simulink model "air_state_hopefully_final"  (R2017b)
settings: Solver=VariableStepAuto  StartTime=0.0  StopTime=10  RelTol=1e-3
settings Model: Creator=benma  LastModifiedBy=benma

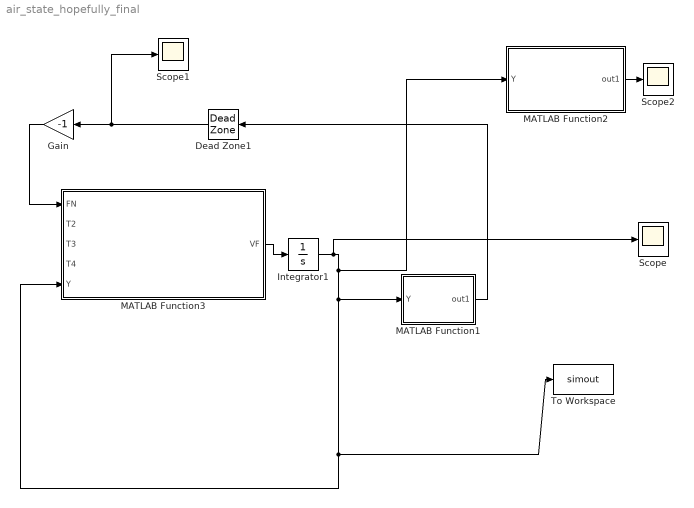
== system air_state_hopefully_final ==
  Dead Zone1 : DeadZone  LowerValue=-inf  UpperValue=0  SaturateOnIntegerOverflow=on
  Gain : Gain  Gain=-1
  Integrator1 : Integrator  InitialCondition=[130 270 80 330 0 0 0 0 0 0]*pi/180  ZeroCross=off
  MATLAB Function1 : MATLAB Function  TreatAsAtomicUnit=on
  MATLAB Function2 : MATLAB Function  TreatAsAtomicUnit=on
  MATLAB Function3 : MATLAB Function  TreatAsAtomicUnit=on
  Scope : Scope
  Scope1 : Scope
  Scope2 : Scope
  To Workspace : ToWorkspace  VariableName=simout  SaveFormat=Timeseries  SampleTime=-1
  wires:
  MATLAB Function2/1(out1) -> Scope2/1
  MATLAB Function3/1(VF) -> Integrator1/1
  Integrator1/1 -> Scope/1, MATLAB Function2/1(Y), MATLAB Function1/1(Y), To Workspace/1, MATLAB Function3/5(Y)
  MATLAB Function1/1(out1) -> Dead Zone1/1
  Dead Zone1/1 -> Scope1/1, Gain/1
  Gain/1 -> MATLAB Function3/1(FN)

== matlab function air_state_hopefully_final/MATLAB Function1 ==
  data: Y input; out1 output
function out1 = ground_force(Y)
%GROUND_FORCE
%    OUT1 = GROUND_FORCE(Y)

%    This function was generated by the Symbolic Math Toolbox version 8.0.
%    22-Oct-2018 11:02:05

if Y(5)<=0
    out1 = -100000*Y(5) - 100*Y(10);
else
    out1 = 0;

% t2 = Y(7);
% t3 = Y(1);
% t4 = Y(2);
% t5 = Y(6);
% t6 = Y(3);
% t7 = Y(8);
% t8 = Y(4);
% t9 = t3+t4+t6+t8;
% t10 = sin(t9);
% t11 = Y(9);
% t12 = t2+t5+t7+t11;
% t13 = t10.*t12.*(1.0./2.0);
% t14 = t3+t4;
% t15 = sin(t14);
% t16 = t2+t5;
% t17 = t15.*t16.*(5.0./2.0);
% t18 = t3+t4+t6; 
% t19 = sin(t18);
% t20 = t2+t5+t7;
% t21 = t19.*t20.*(3.0./2.0);
% out1 = -t7.*(t13+t21)-t5.*(t13+t17+t21+t5.*sin(t3).*(7.0./2.0))-t2.*(t13+t17+t21)-t10.*t11.*t12.*(1.0./2.0)+9.81e2./2.5e1;
end

== matlab function air_state_hopefully_final/MATLAB Function2 ==
  data: Y input; out1 output
function out1 = center_of_mass_state(Y)
%CENTER_OF_MASS_STATE
%    OUT1 = CENTER_OF_MASS_STATE(Y)

%    This function was generated by the Symbolic Math Toolbox version 8.0.
%    22-Oct-2018 12:19:55

t2 = Y(1);
t3 = Y(2);
t4 = Y(3);
t5 = t2+t3;
t6 = Y(4);
t7 = t2+t3+t4+t6;
t8 = t2+t3+t4;
t9 = sin(t2);
t10 = sin(t7);
t11 = Y(6);
t12 = sin(t5);
t13 = Y(7);
t14 = sin(t8);
t15 = Y(8);
t16 = cos(t2);
t17 = cos(t7);
t18 = Y(9);
t19 = t11+t13+t15+t18;
t20 = cos(t5);
t21 = t11+t13;
t22 = cos(t8);
t23 = t11+t13+t15;
out1 = [t16.*(7.0./8.0)+t17.*(1.0./8.0)+t20.*(5.0./8.0)+t22.*(3.0./8.0);t9.*(7.0./8.0)+t10.*(1.0./8.0)+t12.*(5.0./8.0)+t14.*(3.0./8.0)+Y(5);t9.*t11.*(-7.0./8.0)-t10.*t19.*(1.0./8.0)-t12.*t21.*(5.0./8.0)-t14.*t23.*(3.0./8.0);t11.*t16.*(7.0./8.0)+t17.*t19.*(1.0./8.0)+t20.*t21.*(5.0./8.0)+t22.*t23.*(3.0./8.0)+Y(10)];

== matlab function air_state_hopefully_final/MATLAB Function3 ==
  data: FN input; T2 input; VF output; T3 input; T4 input; Y input
function VF = Air_with_force(FN,T2,T3,T4,Y)
%AIR_WITH_FORCE
%    VF = AIR_WITH_FORCE(FN,T2,T3,T4,Y)

%    This function was generated by the Symbolic Math Toolbox version 8.0.
%    27-Oct-2018 21:34:20

t2 = Y(1);
t3 = t2.*2.0;
t4 = Y(2);
t5 = t4.*2.0;
t6 = Y(4);
t7 = Y(3);
t8 = t7.*2.0;
t9 = t6.*2.0;
t10 = Y(6);
t11 = t10.^2;
t12 = t3+t4+t7+t9;
t13 = cos(t12);
t14 = t3+t4;
t15 = sin(t14);
t16 = Y(7);
t17 = t4-t7;
t18 = sin(t17);
t19 = t16.^2;
t20 = Y(8);
t21 = t4+t8;
t22 = sin(t21);
t23 = t4-t9;
t24 = sin(t23);
t25 = t4+t9;
t26 = sin(t25);
t27 = cos(t8);
t28 = cos(t9);
t29 = t3+t4-t7;
t30 = sin(t29);
t31 = t20.^2;
t32 = t3+t4+t8;
t33 = sin(t32);
t34 = t3+t4-t9;
t35 = sin(t34);
t36 = t3+t4+t9;
t37 = sin(t36);
t38 = -t4+t7+t9;
t39 = sin(t38);
t40 = t4+t8+t9;
t41 = sin(t40);
t42 = cos(t14);
t43 = cos(t21);
t44 = cos(t17);
t45 = cos(t23);
t46 = cos(t25);
t47 = t3+t4-t6-t7;
t48 = sin(t47);
t49 = t3+t4-t7-t9;
t50 = sin(t49);
t51 = Y(9);
t52 = t3+t4+t8+t9;
t53 = sin(t52);
t54 = cos(t32);
t55 = cos(t29);
t56 = cos(t34);
t57 = cos(t36);
t58 = cos(t40);
t59 = cos(t38);
t60 = cos(t52);
t61 = cos(t49);
t62 = t3-t8;
t63 = t3+t8;
t64 = t3-t9;
t65 = t3+t9;
t66 = t5+t8;
t67 = t5-t9;
t68 = t5+t9;
t69 = t3+t4+t6+t7;
t70 = sin(t69);
t71 = t51.^2;
t72 = -t3+t8+t9;
t73 = t3+t8+t9;
t74 = t5+t8+t9;
t75 = sin(t4);
t76 = t3+t5;
t77 = cos(t76);
t78 = t8+t9;
t79 = cos(t78);
t80 = t4+t7;
t81 = sin(t80);
t82 = t3+t5+t8;
t83 = cos(t82);
t84 = t3+t5+t9;
t85 = cos(t84);
t86 = cos(t4);
t87 = t3+t4+t7;
t88 = sin(t87);
t89 = -t4+t6+t7;
t90 = sin(t89);
t91 = t4+t6-t7;
t92 = sin(t91);
t93 = t4-t6+t7;
t94 = sin(t93);
t95 = t4+t7+t9;
t96 = sin(t95);
t97 = t3+t5+t8+t9;
t98 = cos(t97);
t99 = cos(t80);
t100 = t3+t4+t6-t7;
t101 = t3+t4-t6+t7;
t102 = sin(t100);
t103 = sin(t101);
t104 = sin(t12);
t105 = cos(t87);
t106 = cos(t95);
t107 = t3+t5-t9;
t108 = cos(t107);
t109 = cos(t72);
t110 = cos(t73);
t111 = cos(t74);
t112 = t98.*3.0;
t113 = cos(t3);
t114 = cos(t5);
t115 = t77.*2.19e2;
t116 = cos(t62);
t117 = t116.*2.43e2;
t118 = cos(t63);
t119 = t118.*2.43e2;
t120 = cos(t64);
t121 = t120.*2.16e2;
t122 = cos(t65);
t123 = t122.*2.16e2;
t124 = cos(t66);
t125 = t124.*8.1e1;
t126 = cos(t67);
t127 = t126.*8.1e1;
t128 = cos(t68);
t129 = t128.*8.1e1;
t130 = t79.*8.1e1;
t131 = sin(t3);
t132 = sin(t5);
t133 = sin(t8);
t134 = T3.*t13.*9.0;
t135 = cos(t100);
t136 = cos(t101);
t137 = T4.*t136.*2.7e1;
t138 = t11.*t18.*1.08e2;
t139 = t3+t7;
t140 = sin(t139);
t141 = t18.*t19.*1.08e2;
t142 = t18.*t31.*1.08e2;
t143 = t5+t7;
t144 = sin(t143);
t145 = -t6+t7;
t146 = sin(t145);
t147 = t7+t9;
t148 = sin(t147);
t149 = t3+t5+t7;
t150 = sin(t149);
t151 = t19.*t33.*(2.7e1./2.0);
t152 = t3+t6-t7;
t153 = sin(t152);
t154 = t19.*t35.*1.8e1;
t155 = t19.*t37.*1.8e1;
t156 = t3-t6+t7;
t157 = sin(t156);
t158 = t11.*t39.*9.0;
t159 = -t3+t7+t9;
t160 = sin(t159);
t161 = t3+t7+t9;
t162 = sin(t161);
t163 = t19.*t39.*9.0;
t164 = t5-t6+t7;
t165 = sin(t164);
t166 = t31.*t39.*9.0;
t167 = t5+t7+t9;
t168 = sin(t167);
t169 = t19.*t41.*3.0;
t170 = t2+t5;
t171 = cos(t170);
t172 = t2-t8;
t173 = cos(t172);
t174 = t2+t8;
t175 = cos(t174);
t176 = t2-t9;
t177 = cos(t176);
t178 = t2+t9;
t179 = cos(t178);
t180 = T3.*t42.*4.11e2;
t181 = T3.*t43.*1.62e2;
t182 = cos(t139);
t183 = T4.*t44.*3.24e2;
t184 = T3.*t45.*8.1e1;
t185 = T3.*t46.*8.1e1;
t186 = cos(t143);
t187 = cos(t147);
t188 = t11.*t50.*(9.0./2.0);
t189 = t3+t5-t6+t7;
t190 = sin(t189);
t191 = t19.*t50.*(9.0./2.0);
t192 = t31.*t50.*(9.0./2.0);
t193 = t3+t5+t7+t9;
t194 = sin(t193);
t195 = t2+t5+t8;
t196 = cos(t195);
t197 = FN.*t196.*2.7e1;
t198 = t2+t5-t9;
t199 = cos(t198);
t200 = FN.*t199.*2.7e1;
t201 = t2+t5+t9;
t202 = cos(t201);
t203 = FN.*t202.*2.7e1;
t204 = t2+t8+t9;
t205 = cos(t204);
t206 = FN.*t205.*9.0;
t207 = T3.*t55.*1.62e2;
t208 = cos(t149);
t209 = T3.*t59.*5.4e1;
t210 = cos(t159);
t211 = cos(t161);
t212 = cos(t167);
t213 = t2+t5+t8+t9;
t214 = cos(t213);
t215 = cos(t47);
t216 = T4.*t215.*3.6e1;
t217 = T3.*t60.*9.0;
t218 = T4.*t61.*2.7e1;
t219 = cos(t193);
t220 = sin(t76);
t221 = t3-t7;
t222 = sin(t221);
t223 = sin(t63);
t224 = sin(t62);
t225 = sin(t64);
t226 = t11.*t225.*3.6e1;
t227 = sin(t65);
t228 = t11.*t227.*3.6e1;
t229 = sin(t66);
t230 = sin(t67);
t231 = sin(t68);
t232 = sin(t78);
t233 = t11.*t70.*(1.0./2.0);
t234 = t19.*t70.*(1.0./2.0);
t235 = t31.*t70.*(1.0./2.0);
t236 = t70.*t71.*(1.0./2.0);
t237 = sin(t107);
t238 = sin(t84);
t239 = sin(t73);
t240 = sin(t72);
t241 = sin(t74);
t242 = t11.*t241.*(3.0./2.0);
t243 = t4+t6+t7;
t244 = cos(t243);
t245 = T4.*t244.*1.8e1;
t246 = t19.*t75.*(6.75e2./2.0);
t247 = sin(t7);
t248 = cos(t221);
t249 = T2.*t79.*2.7e1;
t250 = -t2+t8+t9;
t251 = cos(t250);
t252 = FN.*t251.*9.0;
t253 = cos(t69);
t254 = t11.*t81.*4.5e1;
t255 = t19.*t81.*4.5e1;
t256 = t31.*t81.*4.5e1;
t257 = t6+t7;
t258 = sin(t257);
t259 = T2.*t108.*2.7e1;
t260 = T2.*t85.*2.7e1;
t261 = cos(t2);
t262 = FN.*t261.*4.93e2;
t263 = cos(t7);
t264 = t11.*t92.*2.7e1;
t265 = t11.*t94.*(2.7e1./2.0);
t266 = -t3+t6+t7;
t267 = sin(t266);
t268 = t3+t6+t7;
t269 = sin(t268);
t270 = t19.*t92.*2.7e1;
t271 = t19.*t94.*(2.7e1./2.0);
t272 = t31.*t92.*2.7e1;
t273 = t31.*t94.*(2.7e1./2.0);
t274 = t5+t6+t7;
t275 = sin(t274);
t276 = t71.*t92.*2.7e1;
t277 = t71.*t94.*(2.7e1./2.0);
t278 = T3.*t99.*2.16e2;
t279 = t3+t5+t6+t7;
t280 = t11.*t104.*(3.0./2.0);
t281 = sin(t279);
t282 = t19.*t104.*(3.0./2.0);
t283 = t31.*t104.*(3.0./2.0);
t284 = T4.*t105.*8.1e1;
t285 = cos(t89);
t286 = cos(t91);
t287 = T4.*t286.*1.62e2;
t288 = cos(t93);
t289 = T4.*t106.*2.7e1;
t290 = t10.*t16.*t81.*9.0e1;
t291 = t10.*t20.*t81.*9.0e1;
t292 = t16.*t20.*t81.*9.0e1;
t293 = t10.*t16.*t92.*5.4e1;
t294 = t10.*t16.*t94.*2.7e1;
t295 = t10.*t20.*t92.*5.4e1;
t296 = t10.*t20.*t94.*2.7e1;
t297 = t10.*t51.*t92.*5.4e1;
t298 = t16.*t20.*t92.*5.4e1;
t299 = t10.*t51.*t94.*2.7e1;
t300 = t16.*t20.*t94.*2.7e1;
t301 = t16.*t51.*t92.*5.4e1;
t302 = t16.*t51.*t94.*2.7e1;
t303 = t20.*t51.*t92.*5.4e1;
t304 = t20.*t51.*t94.*2.7e1;
t305 = t10.*t16.*t104.*3.0;
t306 = t10.*t20.*t104.*3.0;
t307 = t16.*t20.*t104.*3.0;
t308 = t10.*t16.*t18.*2.16e2;
t309 = t10.*t18.*t20.*2.16e2;
t310 = t16.*t18.*t20.*2.16e2;
t311 = t10.*t16.*t33.*2.7e1;
t312 = t10.*t16.*t35.*3.6e1;
t313 = t10.*t16.*t37.*3.6e1;
t314 = t10.*t16.*t39.*1.8e1;
t315 = t10.*t20.*t39.*1.8e1;
t316 = t10.*t16.*t41.*6.0;
t317 = t16.*t20.*t39.*1.8e1;
t318 = t10.*t16.*t50.*9.0;
t319 = t10.*t20.*t50.*9.0;
t320 = t16.*t20.*t50.*9.0;
t321 = t10.*t16.*t70;
t322 = t10.*t20.*t70;
t323 = t10.*t51.*t70;
t324 = t16.*t20.*t70;
t325 = t16.*t51.*t70;
t326 = t20.*t51.*t70;
t327 = t10.*t16.*t75.*6.75e2;
t493 = t83.*2.7e1;
t494 = t108.*2.7e1;
t495 = t85.*2.7e1;
t496 = t109.*2.7e1;
t497 = t110.*2.7e1;
t498 = t111.*9.0;
t499 = t113.*1.725e3;
t500 = t114.*6.57e2;
t501 = t27.*7.29e2;
t502 = t28.*6.39e2;
t328 = t112+t115+t117+t119+t121+t123+t125+t127+t129+t130-t493-t494-t495-t496-t497-t498-t499-t500-t501-t502+2.542e3;
t329 = 1.0./t328;
t330 = t11.*t132.*(2.19e2./2.0);
t331 = sin(t9);
t332 = t2+t4+t8+t9;
t333 = cos(t332);
t334 = FN.*t333.*6.0;
t335 = cos(t279);
t336 = T4.*t335.*1.2e1;
t337 = t3+t6;
t338 = sin(t337);
t339 = t11.*t146.*(1.53e2./2.0);
t340 = t5+t6;
t341 = sin(t340);
t342 = t19.*t146.*(1.53e2./2.0);
t343 = t31.*t146.*(1.53e2./2.0);
t344 = t6+t8;
t345 = sin(t344);
t346 = t71.*t146.*(1.53e2./2.0);
t347 = T2.*t113.*7.41e2;
t348 = t11.*t33.*(2.7e1./2.0);
t349 = t11.*t153.*2.7e1;
t350 = t31.*t150.*1.8e1;
t351 = t3+t5+t6;
t352 = sin(t351);
t353 = t19.*t153.*2.7e1;
t354 = t31.*t153.*2.7e1;
t355 = -t3+t6+t8;
t356 = sin(t355);
t357 = t3+t6+t8;
t358 = sin(t357);
t359 = t71.*t153.*2.7e1;
t360 = t31.*t160.*9.0;
t361 = t31.*t162.*9.0;
t362 = t5+t6+t8;
t363 = sin(t362);
t364 = t31.*t168.*(9.0./2.0);
t365 = t2-t4;
t366 = cos(t365);
t367 = T4.*t182.*2.43e2;
t368 = T4.*t186.*1.62e2;
t369 = cos(t145);
t370 = T4.*t187.*1.53e2;
t371 = t11.*t190.*(9.0./2.0);
t372 = t19.*t190.*(9.0./2.0);
t373 = t31.*t190.*(9.0./2.0);
t374 = t3+t5+t6+t8;
t375 = sin(t374);
t376 = t71.*t190.*(9.0./2.0);
t377 = -t2+t4+t8;
t378 = cos(t377);
t379 = FN.*t378.*8.1e1;
t380 = -t2+t4+t9;
t381 = cos(t380);
t382 = FN.*t381.*5.4e1;
t383 = t2-t4+t9;
t384 = cos(t383);
t385 = FN.*t384.*5.4e1;
t386 = T2.*t54.*8.1e1;
t387 = T2.*t56.*5.4e1;
t388 = T2.*t57.*5.4e1;
t389 = T2.*t58.*1.8e1;
t390 = cos(t152);
t391 = T4.*t390.*1.62e2;
t392 = cos(t156);
t393 = T4.*t392.*1.62e2;
t394 = cos(t164);
t395 = T4.*t394.*8.1e1;
t396 = -t2+t4+t8+t9;
t397 = cos(t396);
t398 = cos(t189);
t399 = T4.*t219.*9.0;
t400 = t11.*t220.*(7.3e1./2.0);
t401 = t19.*t220.*(7.3e1./2.0);
t402 = t31.*t222.*(2.43e2./2.0);
t403 = t3-t6;
t404 = sin(t403);
t405 = t11.*t229.*(2.7e1./2.0);
t406 = t5-t6;
t407 = sin(t406);
t408 = t11.*t231.*2.7e1;
t409 = sin(t82);
t410 = t3+t5-t6;
t411 = sin(t410);
t412 = t11.*t240.*(9.0./2.0);
t413 = t19.*t240.*(9.0./2.0);
t414 = t19.*t239.*(9.0./2.0);
t415 = t31.*t247.*(6.93e2./2.0);
t416 = sin(t6);
t417 = T2.*t124.*8.1e1;
t418 = T4.*t248.*2.43e2;
t419 = T3.*t120.*1.08e2;
t420 = T3.*t122.*1.08e2;
t421 = t11.*t258.*(6.1e1./2.0);
t422 = t19.*t258.*(6.1e1./2.0);
t423 = t31.*t258.*(6.1e1./2.0);
t424 = t71.*t258.*(6.1e1./2.0);
t425 = T2.*t83.*2.7e1;
t426 = T3.*t83.*2.7e1;
t427 = T2.*t86.*6.03e2;
t428 = t11.*t88.*(2.7e1./2.0);
t429 = t11.*t96.*(9.0./2.0);
t430 = t2+t4;
t431 = cos(t430);
t432 = FN.*t431.*3.47e2;
t433 = cos(t257);
t434 = T4.*t433.*2.85e2;
t435 = t11.*t281;
t436 = t19.*t281;
t437 = t31.*t281;
t438 = t71.*t281;
t439 = t2+t4+t8;
t440 = cos(t439);
t441 = t2+t4-t9;
t442 = cos(t441);
t443 = t2+t4+t9;
t444 = cos(t443);
t445 = cos(t266);
t446 = cos(t268);
t447 = cos(t274);
t448 = t10.*t16.*t258.*6.1e1;
t449 = t10.*t20.*t258.*6.1e1;
t450 = t10.*t51.*t258.*6.1e1;
t451 = t16.*t20.*t258.*6.1e1;
t452 = t16.*t51.*t258.*6.1e1;
t453 = t20.*t51.*t258.*6.1e1;
t454 = t10.*t16.*t281.*2.0;
t455 = t10.*t20.*t281.*2.0;
t456 = t10.*t51.*t281.*2.0;
t457 = t16.*t20.*t281.*2.0;
t458 = t16.*t51.*t281.*2.0;
t459 = t20.*t51.*t281.*2.0;
t460 = t10.*t16.*t146.*1.53e2;
t461 = t10.*t20.*t146.*1.53e2;
t462 = t10.*t51.*t146.*1.53e2;
t463 = t16.*t20.*t146.*1.53e2;
t464 = t16.*t51.*t146.*1.53e2;
t465 = t20.*t51.*t146.*1.53e2;
t466 = t10.*t20.*t150.*3.6e1;
t467 = t10.*t16.*t153.*5.4e1;
t468 = t16.*t20.*t150.*3.6e1;
t469 = t10.*t20.*t153.*5.4e1;
t470 = t10.*t51.*t153.*5.4e1;
t471 = t16.*t20.*t153.*5.4e1;
t472 = t10.*t20.*t160.*1.8e1;
t473 = t10.*t20.*t162.*1.8e1;
t474 = t16.*t51.*t153.*5.4e1;
t475 = t16.*t20.*t160.*1.8e1;
t476 = t16.*t20.*t162.*1.8e1;
t477 = t10.*t20.*t168.*9.0;
t478 = t20.*t51.*t153.*5.4e1;
t479 = t16.*t20.*t168.*9.0;
t480 = t10.*t16.*t190.*9.0;
t481 = t10.*t20.*t190.*9.0;
t482 = t10.*t51.*t190.*9.0;
t483 = t16.*t20.*t190.*9.0;
t484 = t16.*t51.*t190.*9.0;
t485 = t20.*t51.*t190.*9.0;
t486 = t10.*t16.*t220.*7.3e1;
t487 = t10.*t20.*t222.*2.43e2;
t488 = t16.*t20.*t222.*2.43e2;
t489 = t10.*t16.*t240.*9.0;
t490 = t10.*t16.*t239.*9.0;
t491 = t10.*t20.*t247.*6.93e2;
t492 = t16.*t20.*t247.*6.93e2;
t503 = t11.*t133.*(2.43e2./2.0);
t504 = t19.*t133.*(2.43e2./2.0);
t505 = -t2+t4+t7+t9;
t506 = cos(t505);
t507 = FN.*t506.*9.0;
t508 = t2-t4+t7+t9;
t509 = cos(t508);
t510 = t2+t4-t7-t9;
t511 = cos(t510);
t512 = FN.*t511.*1.8e1;
t513 = T3.*t114.*3.15e2;
t514 = t11.*t39.*1.8e1;
t515 = t11.*t165.*(2.7e1./2.0);
t516 = t19.*t165.*(2.7e1./2.0);
t517 = t11.*t168.*(9.0./2.0);
t518 = t71.*t352.*(2.1e1./2.0);
t519 = t19.*t168.*(9.0./2.0);
t520 = t71.*t356.*(2.7e1./2.0);
t521 = t71.*t358.*(2.7e1./2.0);
t522 = t71.*t363.*(9.0./2.0);
t523 = T2.*t44.*3.24e2;
t524 = cos(t337);
t525 = cos(t340);
t526 = cos(t344);
t527 = T2.*t208.*5.4e1;
t528 = T3.*t208.*5.4e1;
t529 = T2.*t210.*5.4e1;
t530 = T2.*t211.*5.4e1;
t531 = cos(t351);
t532 = T2.*t212.*2.7e1;
t533 = cos(t355);
t534 = T3.*t210.*5.4e1;
t535 = cos(t357);
t536 = T3.*t211.*5.4e1;
t537 = cos(t362);
t538 = T3.*t212.*2.7e1;
t539 = T2.*t61.*2.7e1;
t540 = cos(t374);
t541 = t11.*t222.*(2.43e2./2.0);
t542 = t19.*t222.*(2.43e2./2.0);
t543 = t11.*t224.*(8.1e1./2.0);
t544 = t11.*t223.*(8.1e1./2.0);
t545 = t19.*t224.*(8.1e1./2.0);
t546 = t31.*t223.*(8.1e1./2.0);
t547 = t19.*t229.*(2.7e1./2.0);
t548 = t11.*t230.*2.7e1;
t549 = t71.*t404.*(1.59e2./2.0);
t550 = t31.*t229.*(2.7e1./2.0);
t551 = t11.*t232.*(2.7e1./2.0);
t552 = t71.*t407.*(6.3e1./2.0);
t553 = t19.*t232.*(2.7e1./2.0);
t554 = t11.*t238.*9.0;
t555 = t19.*t238.*9.0;
t556 = t2+t4+t7;
t557 = cos(t556);
t558 = FN.*t557.*3.6e1;
t559 = t71.*t416.*(4.67e2./2.0);
t560 = cos(t403);
t561 = cos(t406);
t562 = T3.*t79.*8.1e1;
t563 = sin(t97);
t564 = t2+t4+t7+t9;
t565 = cos(t564);
t566 = cos(t410);
t567 = T3.*t111.*9.0;
t568 = T4.*t109.*2.7e1;
t569 = T4.*t110.*2.7e1;
t570 = T4.*t111.*9.0;
t571 = T2.*t263.*6.75e2;
t572 = T3.*t263.*6.75e2;
t573 = cos(t6);
t574 = t11.*t102.*(2.7e1./2.0);
t575 = t11.*t103.*(9.0./2.0);
t576 = -t2+t4+t7;
t577 = cos(t576);
t578 = t2-t4+t7;
t579 = cos(t578);
t580 = FN.*t579.*1.62e2;
t581 = t2+t4-t7;
t582 = cos(t581);
t583 = T2.*t105.*8.1e1;
t584 = T2.*t106.*2.7e1;
t585 = t10.*t16.*t133.*2.43e2;
t586 = t10.*t16.*t165.*2.7e1;
t587 = t10.*t51.*t352.*2.1e1;
t588 = t10.*t16.*t168.*9.0;
t589 = t16.*t51.*t352.*2.1e1;
t590 = t10.*t51.*t356.*2.7e1;
t591 = t10.*t51.*t358.*2.7e1;
t592 = t20.*t51.*t352.*2.1e1;
t593 = t16.*t51.*t356.*2.7e1;
t594 = t16.*t51.*t358.*2.7e1;
t595 = t10.*t51.*t363.*9.0;
t596 = t20.*t51.*t356.*2.7e1;
t597 = t20.*t51.*t358.*2.7e1;
t598 = t16.*t51.*t363.*9.0;
t599 = t20.*t51.*t363.*9.0;
t600 = t10.*t16.*t222.*2.43e2;
t601 = t10.*t16.*t224.*8.1e1;
t602 = t10.*t20.*t223.*8.1e1;
t603 = t10.*t16.*t229.*2.7e1;
t604 = t16.*t20.*t223.*8.1e1;
t605 = t10.*t51.*t404.*1.59e2;
t606 = t10.*t20.*t229.*2.7e1;
t607 = t16.*t51.*t404.*1.59e2;
t608 = t16.*t20.*t229.*2.7e1;
t609 = t10.*t51.*t407.*6.3e1;
t610 = t10.*t16.*t232.*2.7e1;
t611 = t20.*t51.*t404.*1.59e2;
t612 = t16.*t51.*t407.*6.3e1;
t613 = t20.*t51.*t407.*6.3e1;
t614 = t10.*t16.*t238.*1.8e1;
t615 = t10.*t51.*t416.*4.67e2;
t616 = t16.*t51.*t416.*4.67e2;
t617 = t20.*t51.*t416.*4.67e2;
t618 = t2-t4+t6-t7;
t619 = cos(t618);
t620 = t2-t4-t6+t7;
t621 = cos(t620);
t622 = t2+t4-t6-t7;
t623 = cos(t622);
t624 = sin(t365);
t625 = t2+t4+t6+t7;
t626 = sin(t625);
t627 = sin(t377);
t628 = sin(t380);
t629 = sin(t383);
t630 = sin(t396);
t631 = cos(t625);
t632 = sin(t556);
t633 = -t2+t4+t6+t7;
t634 = t2-t4+t6+t7;
t635 = t2+t4+t6-t7;
t636 = t2+t4-t6+t7;
t637 = sin(t633);
t638 = sin(t634);
t639 = sin(t635);
t640 = sin(t636);
t641 = sin(t564);
t642 = cos(t633);
t643 = cos(t634);
t644 = cos(t635);
t645 = cos(t636);
t646 = sin(t430);
t647 = sin(t576);
t648 = sin(t578);
t649 = sin(t581);
t650 = sin(t439);
t651 = sin(t441);
t652 = sin(t443);
t653 = sin(t618);
t654 = sin(t620);
t655 = sin(t622);
t656 = sin(t505);
t657 = sin(t508);
t658 = sin(t510);
t659 = sin(t332);
VF = [t10;t16;t20;t51;Y(10);(T2.*3.972e3+t134.*6.0+t137.*6.0+t138.*6.0+t141.*6.0+t142.*6.0+t151.*6.0+t154.*6.0+t155.*6.0+t158.*6.0+t163.*6.0+t166.*6.0+t169.*6.0+t180.*6.0+t181.*6.0+t183.*6.0+t184.*6.0+t185.*6.0+t188.*6.0+t191.*6.0+t192.*6.0+t197.*6.0+t200.*6.0+t203.*6.0+t206.*6.0+t207.*6.0+t209.*6.0+t216.*6.0+t217.*6.0+t218.*6.0+t226.*6.0+t228.*6.0+t233.*6.0+t234.*6.0+t235.*6.0+t236.*6.0+t242.*6.0+t245.*6.0+t246.*6.0+t249.*6.0+t252.*6.0+t254.*6.0+t255.*6.0+t256.*6.0+t259.*6.0+t260.*6.0+t262.*6.0+t264.*6.0+t265.*6.0+t270.*6.0+t271.*6.0+t272.*6.0+t273.*6.0+t276.*6.0+t277.*6.0+t278.*6.0+t280.*6.0+t282.*6.0+t283.*6.0+t284.*6.0+t287.*6.0+t289.*6.0+t290.*6.0+t291.*6.0+t292.*6.0+t293.*6.0+t294.*6.0+t295.*6.0+t296.*6.0+t297.*6.0+t298.*6.0+t299.*6.0+t300.*6.0+t301.*6.0+t302.*6.0+t303.*6.0+t304.*6.0+t305.*6.0+t306.*6.0+t307.*6.0+t308.*6.0+t309.*6.0+t310.*6.0+t311.*6.0+t312.*6.0+t313.*6.0+t314.*6.0+t315.*6.0+t316.*6.0+t317.*6.0+t318.*6.0+t319.*6.0+t320.*6.0+t321.*6.0+t322.*6.0+t323.*6.0+t324.*6.0+t325.*6.0+t326.*6.0+t327.*6.0+t330.*6.0+t348.*6.0+t386.*6.0+t387.*6.0+t388.*6.0+t389.*6.0+t412.*6.0+t425.*6.0+t427.*6.0+t543.*6.0+t544.*6.0-FN.*t171.*1.314e3-FN.*t173.*4.86e2-FN.*t175.*4.86e2-FN.*t177.*3.78e2-FN.*t179.*3.78e2-FN.*t214.*1.8e1-T4.*t13.*5.4e1-T2.*t27.*1.458e3-T2.*t28.*1.026e3-T2.*t42.*2.466e3-T2.*t43.*9.72e2-T2.*t45.*4.86e2-T3.*t44.*1.944e3-T2.*t46.*4.86e2-T3.*t54.*4.86e2-T3.*t56.*3.24e2-T4.*t55.*9.72e2-T3.*t57.*3.24e2-T3.*t58.*1.08e2-T2.*t60.*5.4e1-T4.*t59.*3.24e2-T3.*t61.*1.62e2-T2.*t77.*1.314e3-T3.*t86.*3.618e3-T2.*t98.*1.8e1-T4.*t99.*1.296e3-T3.*t105.*4.86e2-T3.*t106.*1.62e2-T4.*t135.*4.86e2-T4.*t253.*1.8e1-T4.*t285.*4.32e2-T4.*t288.*4.86e2-t11.*t15.*9.03e2-t11.*t22.*1.62e2-t15.*t19.*9.03e2-t11.*t24.*2.43e2-t11.*t26.*2.43e2-t11.*t30.*3.24e2-t19.*t22.*1.62e2-t19.*t24.*2.43e2-t19.*t26.*2.43e2+t11.*t35.*1.08e2+t11.*t37.*1.08e2-t19.*t30.*3.24e2+t11.*t41.*1.8e1-t11.*t48.*1.8e1-t30.*t31.*3.24e2-t11.*t53.*9.0-t19.*t48.*1.8e1-t19.*t53.*9.0-t31.*t48.*1.8e1+t11.*t75.*2.025e3-t11.*t88.*8.1e1-t11.*t90.*3.6e1-t11.*t96.*2.7e1-t19.*t88.*8.1e1-t19.*t90.*3.6e1-t11.*t102.*8.1e1-t11.*t103.*2.7e1-t19.*t96.*2.7e1-t31.*t88.*8.1e1-t48.*t71.*1.8e1-t19.*t102.*8.1e1-t31.*t90.*3.6e1-t19.*t103.*2.7e1-t31.*t96.*2.7e1-t31.*t102.*8.1e1-t31.*t103.*2.7e1-t11.*t131.*1.725e3-t71.*t90.*3.6e1-t71.*t102.*8.1e1-t71.*t103.*2.7e1-t11.*t229.*8.1e1-t11.*t230.*8.1e1-t11.*t231.*8.1e1-t11.*t239.*2.7e1-t10.*t15.*t16.*1.806e3-t10.*t16.*t22.*3.24e2-t10.*t16.*t24.*4.86e2-t10.*t16.*t26.*4.86e2-t10.*t16.*t30.*6.48e2-t10.*t20.*t30.*6.48e2-t16.*t20.*t30.*6.48e2-t10.*t16.*t48.*3.6e1-t10.*t20.*t48.*3.6e1-t10.*t16.*t53.*1.8e1-t16.*t20.*t48.*3.6e1-t10.*t48.*t51.*3.6e1-t10.*t16.*t88.*1.62e2-t16.*t48.*t51.*3.6e1-t10.*t16.*t90.*7.2e1-t10.*t20.*t88.*1.62e2-t20.*t48.*t51.*3.6e1-t10.*t20.*t90.*7.2e1-t10.*t16.*t96.*5.4e1-t16.*t20.*t88.*1.62e2-t10.*t20.*t96.*5.4e1-t16.*t20.*t90.*7.2e1-t10.*t16.*t102.*1.62e2-t10.*t16.*t103.*5.4e1-t10.*t20.*t102.*1.62e2-t16.*t20.*t96.*5.4e1-t10.*t20.*t103.*5.4e1-t16.*t20.*t102.*1.62e2-t16.*t20.*t103.*5.4e1-t10.*t51.*t90.*7.2e1-t16.*t51.*t90.*7.2e1-t20.*t51.*t90.*7.2e1-t10.*t51.*t102.*1.62e2-t10.*t51.*t103.*5.4e1-t16.*t51.*t102.*1.62e2-t16.*t51.*t103.*5.4e1-t20.*t51.*t102.*1.62e2-t20.*t51.*t103.*5.4e1)./(t27.*-7.29e2-t28.*6.39e2-t83.*2.7e1-t85.*2.7e1-t109.*2.7e1-t110.*2.7e1-t111.*9.0+t112-t113.*1.725e3-t114.*6.57e2+t115+t117+t119+t121+t123+t125+t127+t129+t130-cos(t3+t5-t6.*2.0).*2.7e1+2.542e3);t329.*(T2.*-1.6e3+T3.*9.38e2-t134-t137-t138-t141-t142-t151-t154-t155-t158-t163-t166-t169-t180-t181-t183-t184-t185-t188-t191-t192-t197-t200-t203-t206-t207-t209-t216-t217-t218-t226-t228-t233-t234-t235-t236-t242-t245-t246-t249-t252-t254-t255-t256-t259-t260-t262-t264-t265-t270-t271-t272-t273-t276-t277-t278-t280-t282-t283-t284-t287-t289-t290-t291-t292-t293-t294-t295-t296-t297-t298-t299-t300-t301-t302-t303-t304-t305-t306-t307-t308-t309-t310-t311-t312-t313-t314-t315-t316-t317-t318-t319-t320-t321-t322-t323-t324-t325-t326-t327+t334+t336+t339+t342+t343+t346+t347+t349+t350+t353+t354+t359+t360+t361+t364+t367+t368+t370+t371+t372+t373+t376+t379+t382+t385+t391+t393+t395+t399+t400+t401+t402+t405+t408+t413+t414+t415+t417+t418+t419+t420+t421+t422+t423+t424+t426+t428+t429+t432+t434+t435+t436+t437+t438+t448+t449+t450+t451+t452+t453+t454+t455+t456+t457+t458+t459+t460+t461+t462+t463+t464+t465+t466+t467+t468+t469+t470+t471+t472+t473+t474+t475+t476+t477+t478+t479+t480+t481+t482+t483+t484+t485+t486+t487+t488+t489+t490+t491+t492+t503+t504+t517+t519+t528+t534+t536+t538+t541+t542+t545+t548+t567+t572+t574+t575+t585+t588+t600+t601+FN.*t171.*2.19e2+FN.*t173.*8.1e1+FN.*t175.*8.1e1+FN.*t177.*6.3e1+FN.*t179.*6.3e1+FN.*t214.*3.0-FN.*t366.*4.11e2-FN.*t397.*9.0-FN.*t440.*5.4e1-FN.*t442.*4.5e1-FN.*t444.*4.5e1+T4.*t13.*9.0+T2.*t27.*2.43e2+T2.*t28.*4.5e2-T3.*t28.*2.79e2+T2.*t42.*8.22e2+T2.*t43.*3.24e2+T2.*t45.*1.62e2+T3.*t44.*3.24e2+T2.*t46.*1.62e2-T2.*t54.*1.62e2+T3.*t54.*8.1e1-T2.*t56.*1.08e2-T2.*t57.*1.08e2+T3.*t56.*5.4e1+T4.*t55.*1.62e2-T2.*t58.*3.6e1+T3.*t57.*5.4e1+T3.*t58.*1.8e1+T2.*t60.*1.8e1+T4.*t59.*5.4e1+T3.*t61.*2.7e1+T2.*t77.*2.19e2-T2.*t83.*5.4e1-T2.*t86.*1.206e3+T3.*t86.*6.03e2+T2.*t98.*6.0-T3.*t98.*3.0+T4.*t99.*2.16e2+T3.*t105.*8.1e1+T3.*t106.*2.7e1-T2.*t111.*9.0-T3.*t113.*7.41e2-T2.*t120.*1.08e2-T2.*t122.*1.08e2-T3.*t124.*8.1e1+T4.*t135.*8.1e1-T3.*t182.*2.43e2-T3.*t186.*1.62e2-T3.*t187.*1.53e2-T4.*t208.*5.4e1-T4.*t210.*5.4e1-T4.*t211.*5.4e1-T4.*t212.*2.7e1-T3.*t219.*9.0-T3.*t248.*2.43e2+T4.*t253.*3.0-T4.*t263.*6.75e2+T4.*t285.*7.2e1+T4.*t288.*8.1e1-T4.*t369.*4.59e2-T4.*t398.*2.7e1-T4.*t445.*9.9e1-T4.*t446.*9.9e1-T4.*t447.*3.6e1+t11.*t15.*2.19e2+t11.*t22.*8.1e1+t15.*t19.*(3.01e2./2.0)+t11.*t24.*8.1e1+t11.*t26.*8.1e1+t11.*t30.*5.4e1+t19.*t22.*2.7e1+t19.*t24.*(8.1e1./2.0)-t11.*t33.*2.7e1+t19.*t26.*(8.1e1./2.0)-t11.*t35.*2.7e1-t11.*t37.*2.7e1+t19.*t30.*5.4e1-t11.*t41.*9.0+t11.*t48.*3.0+t30.*t31.*5.4e1+t11.*t53.*3.0+t19.*t48.*3.0+t19.*t53.*(3.0./2.0)+t31.*t48.*3.0-t11.*t75.*6.48e2+t11.*t90.*6.0+t19.*t88.*(2.7e1./2.0)+t19.*t90.*6.0+t19.*t96.*(9.0./2.0)+t31.*t88.*(2.7e1./2.0)+t48.*t71.*3.0+t19.*t102.*(2.7e1./2.0)+t31.*t90.*6.0+t19.*t103.*(9.0./2.0)+t31.*t96.*(9.0./2.0)+t31.*t102.*(2.7e1./2.0)+t31.*t103.*(9.0./2.0)+t11.*t131.*(5.75e2./2.0)-t11.*t132.*2.19e2-t11.*t140.*(2.43e2./2.0)-t19.*t132.*(2.19e2./2.0)-t11.*t144.*5.4e1-t11.*t148.*(5.1e1./2.0)-t19.*t140.*(2.43e2./2.0)+t11.*t150.*1.8e1+t71.*t90.*6.0-t19.*t144.*5.4e1-t19.*t148.*(5.1e1./2.0)-t11.*t157.*2.7e1+t19.*t150.*1.8e1+t11.*t160.*9.0-t31.*t140.*(2.43e2./2.0)+t11.*t162.*9.0+t71.*t102.*(2.7e1./2.0)+t71.*t103.*(9.0./2.0)-t31.*t144.*5.4e1-t11.*t165.*(2.7e1./2.0)-t19.*t157.*2.7e1+t19.*t160.*9.0-t31.*t148.*(5.1e1./2.0)+t19.*t162.*9.0-t19.*t165.*(2.7e1./2.0)-t31.*t157.*2.7e1-t31.*t165.*(2.7e1./2.0)-t11.*t194.*(3.0./2.0)-t19.*t194.*(3.0./2.0)-t31.*t194.*(3.0./2.0)-t71.*t157.*2.7e1-t11.*t223.*8.1e1-t71.*t165.*(2.7e1./2.0)-t19.*t223.*(8.1e1./2.0)-t11.*t232.*(2.7e1./2.0)-t11.*t237.*(9.0./2.0)-t11.*t238.*(9.0./2.0)+t19.*t230.*(2.7e1./2.0)+t11.*t239.*9.0+t19.*t231.*(2.7e1./2.0)-t19.*t232.*(2.7e1./2.0)-t19.*t237.*(9.0./2.0)-t19.*t238.*(9.0./2.0)+t11.*t247.*(6.93e2./2.0)+t19.*t247.*(6.93e2./2.0)-t11.*t267.*(2.1e1./2.0)-t11.*t269.*(2.1e1./2.0)-t11.*t275.*3.0-t19.*t267.*(2.1e1./2.0)-t19.*t269.*(2.1e1./2.0)-t19.*t275.*3.0-t31.*t267.*(2.1e1./2.0)-t31.*t269.*(2.1e1./2.0)-t31.*t275.*3.0-t71.*t267.*(2.1e1./2.0)-t71.*t269.*(2.1e1./2.0)-t71.*t275.*3.0+t10.*t15.*t16.*3.01e2+t10.*t16.*t22.*5.4e1+t10.*t16.*t24.*8.1e1+t10.*t16.*t26.*8.1e1+t10.*t16.*t30.*1.08e2+t10.*t20.*t30.*1.08e2+t16.*t20.*t30.*1.08e2+t10.*t16.*t48.*6.0+t10.*t20.*t48.*6.0+t10.*t16.*t53.*3.0+t16.*t20.*t48.*6.0+t10.*t48.*t51.*6.0+t10.*t16.*t88.*2.7e1+t16.*t48.*t51.*6.0+t10.*t16.*t90.*1.2e1+t10.*t20.*t88.*2.7e1+t20.*t48.*t51.*6.0+t10.*t20.*t90.*1.2e1+t10.*t16.*t96.*9.0+t16.*t20.*t88.*2.7e1+t10.*t20.*t96.*9.0+t16.*t20.*t90.*1.2e1+t10.*t16.*t102.*2.7e1+t10.*t16.*t103.*9.0+t10.*t20.*t102.*2.7e1+t16.*t20.*t96.*9.0+t10.*t20.*t103.*9.0+t16.*t20.*t102.*2.7e1+t16.*t20.*t103.*9.0+t10.*t51.*t90.*1.2e1+t16.*t51.*t90.*1.2e1-t10.*t16.*t132.*2.19e2+t20.*t51.*t90.*1.2e1+t10.*t51.*t102.*2.7e1+t10.*t51.*t103.*9.0-t10.*t16.*t140.*2.43e2+t16.*t51.*t102.*2.7e1-t10.*t16.*t144.*1.08e2-t10.*t20.*t140.*2.43e2+t16.*t51.*t103.*9.0+t20.*t51.*t102.*2.7e1-t10.*t16.*t148.*5.1e1-t10.*t20.*t144.*1.08e2+t20.*t51.*t103.*9.0+t10.*t16.*t150.*3.6e1-t16.*t20.*t140.*2.43e2-t10.*t20.*t148.*5.1e1-t16.*t20.*t144.*1.08e2-t10.*t16.*t157.*5.4e1-t16.*t20.*t148.*5.1e1+t10.*t16.*t160.*1.8e1-t10.*t20.*t157.*5.4e1+t10.*t16.*t162.*1.8e1-t10.*t16.*t165.*2.7e1-t16.*t20.*t157.*5.4e1-t10.*t20.*t165.*2.7e1-t16.*t20.*t165.*2.7e1-t10.*t51.*t157.*5.4e1-t10.*t16.*t194.*3.0-t10.*t20.*t194.*3.0-t16.*t51.*t157.*5.4e1-t10.*t51.*t165.*2.7e1-t20.*t51.*t157.*5.4e1-t16.*t20.*t194.*3.0-t16.*t51.*t165.*2.7e1-t20.*t51.*t165.*2.7e1-t10.*t16.*t223.*8.1e1+t10.*t16.*t230.*2.7e1+t10.*t16.*t231.*2.7e1-t10.*t16.*t232.*2.7e1-t10.*t16.*t237.*9.0-t10.*t16.*t238.*9.0+t10.*t16.*t247.*6.93e2-t10.*t16.*t267.*2.1e1-t10.*t16.*t269.*2.1e1-t10.*t20.*t267.*2.1e1-t10.*t20.*t269.*2.1e1-t10.*t16.*t275.*6.0-t16.*t20.*t267.*2.1e1-t10.*t20.*t275.*6.0-t16.*t20.*t269.*2.1e1-t16.*t20.*t275.*6.0-t10.*t51.*t267.*2.1e1-t10.*t51.*t269.*2.1e1-t16.*t51.*t267.*2.1e1-t10.*t51.*t275.*6.0-t16.*t51.*t269.*2.1e1-t20.*t51.*t267.*2.1e1-t20.*t51.*t269.*2.1e1-t16.*t51.*t275.*6.0-t20.*t51.*t275.*6.0).*6.0;t329.*(T2.*9.38e2-T3.*1.96e3+T4.*1.022e3+t138+t188+t226-t228-t254-t280+t330-t334-t336-t339-t342-t343-t346-t347+t348-t349-t350-t353-t354-t359-t360-t361-t364-t367-t368-t370-t371-t372-t373-t376-t379-t382-t385+t386+t387+t388+t389-t391-t393-t395-t399-t400-t401-t402+t405-t408-t412-t413-t414-t415-t417-t418-t419-t420-t421-t422-t423-t424+t425-t426+t427+t428+t429-t432-t434-t435-t436-t437-t438-t448-t449-t450-t451-t452-t453-t454-t455-t456-t457-t458-t459-t460-t461-t462-t463-t464-t465-t466-t467-t468-t469-t470-t471-t472-t473-t474-t475-t476-t477-t478-t479-t480-t481-t482-t483-t484-t485-t486-t487-t488-t489-t490-t491-t492+t507+t512+t513+t514+t515+t516+t518+t520+t521+t522+t523+t527+t529+t530+t532+t539+t546+t547+t549+t550+t551+t552+t553+t554+t555+t558+t559+t562+t568+t569+t570+t571+t580+t583+t584+t586+t587+t589+t590+t591+t592+t593+t594+t595+t596+t597+t598+t599+t602+t603+t604+t605+t606+t607+t608+t609+t610+t611+t612+t613+t614+t615+t616+t617+FN.*t366.*4.11e2+FN.*t397.*9.0+FN.*t440.*5.4e1+FN.*t442.*4.5e1+FN.*t444.*4.5e1-FN.*t509.*2.7e1-FN.*t565.*3.0-FN.*t577.*8.1e1-FN.*t582.*1.08e2-T2.*t13.*9.0-T2.*t28.*2.79e2+T3.*t28.*2.79e2-T2.*t42.*4.11e2-T2.*t43.*1.62e2-T2.*t45.*8.1e1-T2.*t46.*8.1e1-T2.*t55.*1.62e2-T2.*t59.*5.4e1-T2.*t60.*9.0-T3.*t77.*1.05e2+T4.*t77.*1.05e2-T4.*t79.*8.1e1-T2.*t98.*3.0-T2.*t99.*2.16e2+T3.*t98.*6.0-T4.*t98.*3.0-T3.*t109.*2.7e1+T2.*t111.*9.0-T3.*t110.*2.7e1-T3.*t111.*1.8e1+T3.*t113.*1.446e3-T4.*t113.*7.05e2-T4.*t114.*3.15e2+T2.*t120.*1.08e2+T2.*t122.*1.08e2+T3.*t124.*8.1e1-T2.*t182.*2.43e2+T3.*t182.*4.86e2-T2.*t186.*1.62e2-T2.*t187.*1.53e2+T3.*t186.*3.24e2+T3.*t187.*3.06e2-T3.*t208.*1.08e2+T4.*t208.*5.4e1-T3.*t210.*1.08e2-T3.*t211.*1.08e2+T4.*t210.*5.4e1-T3.*t212.*5.4e1+T4.*t211.*5.4e1+T4.*t212.*2.7e1-T2.*t219.*9.0+T3.*t219.*1.8e1-T2.*t248.*2.43e2+T3.*t248.*4.86e2-T3.*t263.*1.35e3+T4.*t263.*6.75e2+T4.*t369.*4.59e2+T4.*t398.*2.7e1+T4.*t445.*9.9e1+T4.*t446.*9.9e1+T4.*t447.*3.6e1-T4.*t524.*3.33e2-T4.*t525.*1.35e2-T4.*t526.*2.43e2+T4.*t531.*4.5e1+T4.*t533.*8.1e1+T4.*t535.*8.1e1+T4.*t537.*2.7e1-T4.*t540.*9.0-T4.*t560.*3.33e2-T4.*t561.*1.35e2+T4.*t566.*4.5e1+T4.*t573.*9.75e2-t11.*t15.*(1.37e2./2.0)-t11.*t22.*5.4e1-t11.*t24.*(8.1e1./2.0)-t11.*t26.*(8.1e1./2.0)-t11.*t30.*2.7e1+t11.*t35.*9.0+t11.*t37.*9.0+t11.*t41.*6.0-t11.*t53.*(3.0./2.0)+t11.*t75.*(6.21e2./2.0)-t11.*t133.*2.43e2+t11.*t140.*2.43e2+t19.*t132.*(2.19e2./2.0)-t19.*t133.*2.43e2+t11.*t144.*8.1e1+t11.*t148.*8.1e1+t19.*t140.*2.43e2-t11.*t150.*2.7e1+t19.*t144.*8.1e1-t31.*t133.*(2.43e2./2.0)+t19.*t148.*8.1e1+t11.*t157.*2.7e1-t19.*t150.*2.7e1-t11.*t160.*2.7e1+t31.*t140.*(2.43e2./2.0)-t11.*t162.*2.7e1+t31.*t144.*5.4e1+t19.*t157.*2.7e1-t11.*t168.*9.0-t19.*t160.*2.7e1+t31.*t148.*(5.1e1./2.0)-t19.*t162.*2.7e1-t19.*t168.*9.0+t31.*t157.*2.7e1+t31.*t165.*(2.7e1./2.0)+t11.*t194.*3.0+t19.*t194.*3.0+t31.*t194.*(3.0./2.0)+t71.*t157.*2.7e1-t11.*t222.*2.43e2+t11.*t223.*8.1e1-t11.*t224.*8.1e1+t71.*t165.*(2.7e1./2.0)-t19.*t222.*2.43e2+t19.*t223.*8.1e1-t19.*t224.*8.1e1+t19.*t225.*3.6e1-t19.*t227.*3.6e1-t11.*t239.*(9.0./2.0)-t19.*t231.*2.7e1-t31.*t224.*(8.1e1./2.0)+t31.*t225.*3.6e1-t11.*t247.*7.2e2-t31.*t227.*3.6e1+t31.*t230.*(2.7e1./2.0)-t31.*t231.*(2.7e1./2.0)-t19.*t247.*7.2e2-t31.*t237.*(9.0./2.0)+t31.*t238.*(9.0./2.0)+t11.*t267.*(2.1e1./2.0)+t11.*t269.*(2.1e1./2.0)+t11.*t275.*3.0+t19.*t267.*(2.1e1./2.0)+t19.*t269.*(2.1e1./2.0)+t19.*t275.*3.0+t31.*t267.*(2.1e1./2.0)+t31.*t269.*(2.1e1./2.0)+t31.*t275.*3.0+t71.*t267.*(2.1e1./2.0)+t71.*t269.*(2.1e1./2.0)+t11.*t331.*(2.13e2./2.0)+t71.*t275.*3.0-t11.*t338.*(1.59e2./2.0)+t19.*t331.*(2.13e2./2.0)-t11.*t341.*(6.3e1./2.0)-t11.*t345.*(8.1e1./2.0)-t19.*t338.*(1.59e2./2.0)-t19.*t341.*(6.3e1./2.0)+t31.*t331.*(2.13e2./2.0)+t11.*t352.*(2.1e1./2.0)-t19.*t345.*(8.1e1./2.0)+t11.*t356.*(2.7e1./2.0)+t11.*t358.*(2.7e1./2.0)-t31.*t338.*(1.59e2./2.0)+t19.*t352.*(2.1e1./2.0)-t31.*t341.*(6.3e1./2.0)+t11.*t363.*(9.0./2.0)+t19.*t356.*(2.7e1./2.0)-t31.*t345.*(8.1e1./2.0)+t19.*t358.*(2.7e1./2.0)+t19.*t363.*(9.0./2.0)+t31.*t352.*(2.1e1./2.0)-t11.*t375.*(3.0./2.0)+t31.*t356.*(2.7e1./2.0)+t31.*t358.*(2.7e1./2.0)-t19.*t375.*(3.0./2.0)+t31.*t363.*(9.0./2.0)-t31.*t375.*(3.0./2.0)-t71.*t338.*(1.59e2./2.0)-t71.*t341.*(6.3e1./2.0)+t11.*t404.*(1.59e2./2.0)-t71.*t345.*(8.1e1./2.0)+t11.*t407.*(6.3e1./2.0)-t11.*t409.*(9.0./2.0)-t11.*t411.*(2.1e1./2.0)+t19.*t404.*(1.59e2./2.0)+t19.*t407.*(6.3e1./2.0)+t11.*t416.*(4.67e2./2.0)-t19.*t409.*(9.0./2.0)-t19.*t411.*(2.1e1./2.0)+t19.*t416.*(4.67e2./2.0)+t31.*t404.*(1.59e2./2.0)+t31.*t407.*(6.3e1./2.0)-t31.*t409.*(9.0./2.0)-t31.*t411.*(2.1e1./2.0)-t71.*t375.*(3.0./2.0)+t31.*t416.*(4.67e2./2.0)-t71.*t411.*(2.1e1./2.0)+t10.*t16.*t132.*2.19e2-t10.*t16.*t133.*4.86e2-t10.*t20.*t133.*2.43e2+t10.*t16.*t140.*4.86e2-t16.*t20.*t133.*2.43e2+t10.*t16.*t144.*1.62e2+t10.*t20.*t140.*2.43e2+t10.*t16.*t148.*1.62e2+t10.*t20.*t144.*1.08e2-t10.*t16.*t150.*5.4e1+t16.*t20.*t140.*2.43e2+t10.*t20.*t148.*5.1e1+t16.*t20.*t144.*1.08e2+t10.*t16.*t157.*5.4e1+t16.*t20.*t148.*5.1e1-t10.*t16.*t160.*5.4e1+t10.*t20.*t157.*5.4e1-t10.*t16.*t162.*5.4e1+t16.*t20.*t157.*5.4e1-t10.*t16.*t168.*1.8e1+t10.*t20.*t165.*2.7e1+t16.*t20.*t165.*2.7e1+t10.*t51.*t157.*5.4e1+t10.*t16.*t194.*6.0+t10.*t20.*t194.*3.0+t16.*t51.*t157.*5.4e1+t10.*t51.*t165.*2.7e1+t20.*t51.*t157.*5.4e1+t16.*t20.*t194.*3.0+t16.*t51.*t165.*2.7e1+t20.*t51.*t165.*2.7e1-t10.*t16.*t222.*4.86e2+t10.*t16.*t223.*1.62e2-t10.*t16.*t224.*1.62e2+t10.*t16.*t225.*7.2e1-t10.*t16.*t227.*7.2e1-t10.*t20.*t224.*8.1e1+t10.*t20.*t225.*7.2e1-t10.*t16.*t231.*5.4e1-t10.*t20.*t227.*7.2e1+t10.*t20.*t230.*2.7e1-t16.*t20.*t224.*8.1e1-t10.*t20.*t231.*2.7e1+t16.*t20.*t225.*7.2e1-t16.*t20.*t227.*7.2e1+t16.*t20.*t230.*2.7e1-t10.*t20.*t237.*9.0-t16.*t20.*t231.*2.7e1+t10.*t20.*t238.*9.0-t10.*t16.*t247.*1.44e3-t16.*t20.*t237.*9.0+t16.*t20.*t238.*9.0+t10.*t16.*t267.*2.1e1+t10.*t16.*t269.*2.1e1+t10.*t20.*t267.*2.1e1+t10.*t20.*t269.*2.1e1+t10.*t16.*t275.*6.0+t16.*t20.*t267.*2.1e1+t10.*t20.*t275.*6.0+t16.*t20.*t269.*2.1e1+t16.*t20.*t275.*6.0+t10.*t51.*t267.*2.1e1+t10.*t51.*t269.*2.1e1+t16.*t51.*t267.*2.1e1+t10.*t51.*t275.*6.0+t16.*t51.*t269.*2.1e1+t20.*t51.*t267.*2.1e1+t20.*t51.*t269.*2.1e1+t16.*t51.*t275.*6.0+t20.*t51.*t275.*6.0+t10.*t16.*t331.*2.13e2+t10.*t20.*t331.*2.13e2-t10.*t16.*t338.*1.59e2-t10.*t16.*t341.*6.3e1+t16.*t20.*t331.*2.13e2-t10.*t20.*t338.*1.59e2-t10.*t16.*t345.*8.1e1-t10.*t20.*t341.*6.3e1-t16.*t20.*t338.*1.59e2-t10.*t20.*t345.*8.1e1-t16.*t20.*t341.*6.3e1+t10.*t16.*t352.*2.1e1-t16.*t20.*t345.*8.1e1+t10.*t16.*t356.*2.7e1+t10.*t20.*t352.*2.1e1+t10.*t16.*t358.*2.7e1+t10.*t20.*t356.*2.7e1+t10.*t20.*t358.*2.7e1+t16.*t20.*t352.*2.1e1+t10.*t16.*t363.*9.0+t16.*t20.*t356.*2.7e1+t10.*t20.*t363.*9.0+t16.*t20.*t358.*2.7e1-t10.*t51.*t338.*1.59e2+t16.*t20.*t363.*9.0-t10.*t16.*t375.*3.0-t10.*t51.*t341.*6.3e1-t10.*t20.*t375.*3.0-t16.*t51.*t338.*1.59e2-t10.*t51.*t345.*8.1e1-t16.*t51.*t341.*6.3e1-t20.*t51.*t338.*1.59e2-t16.*t20.*t375.*3.0-t16.*t51.*t345.*8.1e1-t20.*t51.*t341.*6.3e1-t20.*t51.*t345.*8.1e1+t10.*t16.*t404.*1.59e2+t10.*t16.*t407.*6.3e1+t10.*t20.*t404.*1.59e2-t10.*t16.*t409.*9.0-t10.*t51.*t375.*3.0-t10.*t16.*t411.*2.1e1+t10.*t20.*t407.*6.3e1-t10.*t20.*t409.*9.0+t16.*t20.*t404.*1.59e2-t10.*t20.*t411.*2.1e1+t10.*t16.*t416.*4.67e2-t16.*t51.*t375.*3.0+t16.*t20.*t407.*6.3e1-t16.*t20.*t409.*9.0+t10.*t20.*t416.*4.67e2-t20.*t51.*t375.*3.0-t16.*t20.*t411.*2.1e1+t16.*t20.*t416.*4.67e2-t10.*t51.*t411.*2.1e1-t16.*t51.*t411.*2.1e1-t20.*t51.*t411.*2.1e1).*6.0;t329.*(T3.*-1.022e3+T4.*3.25e3+t138+t188-t233+t242-t254-t265-t280-t371-t372+t405-t408+t412+t413+t414+t428+t429-t480+t489+t490-t503-t504+t507+t512+t513+t514+t515+t516-t517+t518-t519+t520+t521+t522+t523+t527-t528+t529+t530+t532-t534-t536-t538+t539-t541-t542-t543+t544-t545+t546+t547+t548+t549+t550-t551+t552-t553+t554+t555+t558+t559+t562-t567+t568+t569+t570+t571-t572-t574+t575+t580+t583+t584-t585+t586+t587-t588+t589+t590+t591+t592+t593+t594+t595+t596+t597+t598+t599-t600-t601+t602+t603+t604+t605+t606+t607+t608+t609-t610+t611+t612+t613+t614+t615+t616+t617-FN.*t509.*2.7e1-FN.*t565.*3.0-FN.*t577.*8.1e1-FN.*t582.*1.08e2-FN.*t619.*2.7e1+FN.*t621.*8.1e1+FN.*t623.*2.4e1+FN.*t631.*2.0+FN.*t642.*3.0-FN.*t643.*3.6e1-FN.*t644.*5.4e1+FN.*t645.*9.0-T2.*t13.*9.0-T4.*t27.*7.29e2-T2.*t55.*1.62e2-T2.*t59.*5.4e1-T3.*t77.*1.05e2+T4.*t77.*3.0e2-T4.*t79.*8.1e1-T4.*t83.*2.7e1-T2.*t99.*2.16e2+T3.*t98.*3.0-T4.*t98.*3.0-T3.*t109.*2.7e1-T3.*t110.*2.7e1+T3.*t113.*7.05e2-T4.*t113.*2.22e3-T4.*t114.*9.0e2+T4.*t116.*2.43e2+T4.*t118.*2.43e2+T4.*t124.*8.1e1-T2.*t135.*8.1e1+T2.*t136.*2.7e1-T2.*t182.*2.43e2+T3.*t182.*2.43e2-T2.*t186.*1.62e2-T2.*t187.*1.53e2+T3.*t186.*1.62e2+T3.*t187.*1.53e2+T2.*t215.*3.6e1-T2.*t219.*9.0+T3.*t219.*9.0+T2.*t244.*1.8e1-T2.*t248.*2.43e2+T3.*t248.*2.43e2-T2.*t253.*3.0-T2.*t285.*7.2e1+T2.*t286.*1.62e2-T2.*t288.*8.1e1-T2.*t335.*1.2e1+T3.*t335.*1.2e1+T2.*t369.*4.59e2-T3.*t369.*4.59e2-T2.*t390.*1.62e2+T3.*t390.*1.62e2-T2.*t392.*1.62e2+T3.*t392.*1.62e2-T2.*t394.*8.1e1+T3.*t394.*8.1e1+T2.*t398.*2.7e1-T3.*t398.*2.7e1-T2.*t433.*2.85e2+T3.*t433.*2.85e2+T2.*t445.*9.9e1+T2.*t446.*9.9e1-T3.*t445.*9.9e1+T2.*t447.*3.6e1-T3.*t446.*9.9e1-T3.*t447.*3.6e1+T3.*t524.*3.33e2+T3.*t525.*1.35e2-T4.*t524.*6.66e2+T3.*t526.*2.43e2-T4.*t525.*2.7e2-T4.*t526.*4.86e2-T3.*t531.*4.5e1+T4.*t531.*9.0e1-T3.*t533.*8.1e1+T4.*t533.*1.62e2-T3.*t535.*8.1e1+T4.*t535.*1.62e2-T3.*t537.*2.7e1+T4.*t537.*5.4e1+T3.*t540.*9.0-T4.*t540.*1.8e1+T3.*t560.*3.33e2+T3.*t561.*1.35e2-T4.*t560.*6.66e2-T4.*t561.*2.7e2-T3.*t566.*4.5e1+T4.*t566.*9.0e1-T3.*t573.*9.75e2+T4.*t573.*1.95e3-t11.*t30.*2.7e1+t11.*t48.*6.0+t11.*t90.*2.4e1+t11.*t92.*5.4e1+t11.*t140.*(2.43e2./2.0)+t11.*t144.*2.7e1-t11.*t146.*(3.33e2./2.0)+t11.*t148.*(1.11e2./2.0)+t19.*t140.*(2.43e2./2.0)-t11.*t150.*9.0+t19.*t144.*2.7e1-t11.*t153.*5.4e1-t31.*t133.*(2.43e2./2.0)-t19.*t146.*(3.33e2./2.0)+t19.*t148.*(1.11e2./2.0)+t11.*t157.*5.4e1-t19.*t150.*9.0-t11.*t160.*1.8e1-t19.*t153.*5.4e1-t11.*t162.*1.8e1+t19.*t157.*5.4e1-t19.*t160.*1.8e1-t19.*t162.*1.8e1+t11.*t194.*(3.0./2.0)+t19.*t194.*(3.0./2.0)+t11.*t225.*7.2e1-t11.*t227.*7.2e1+t19.*t223.*(8.1e1./2.0)+t19.*t225.*7.2e1-t19.*t227.*7.2e1-t11.*t237.*9.0+t19.*t230.*2.7e1+t11.*t239.*(9.0./2.0)-t19.*t231.*2.7e1-t31.*t224.*(8.1e1./2.0)-t19.*t237.*9.0+t31.*t225.*7.2e1-t11.*t247.*(7.47e2./2.0)-t31.*t227.*7.2e1+t19.*t241.*(3.0./2.0)+t31.*t230.*2.7e1-t31.*t231.*2.7e1-t31.*t232.*(2.7e1./2.0)-t19.*t247.*(7.47e2./2.0)-t31.*t237.*9.0+t11.*t258.*(1.21e2./2.0)+t31.*t238.*9.0+t31.*t239.*(9.0./2.0)+t31.*t240.*(9.0./2.0)+t31.*t241.*(3.0./2.0)+t19.*t258.*(1.21e2./2.0)-t11.*t267.*(3.9e1./2.0)-t11.*t269.*(3.9e1./2.0)-t11.*t275.*6.0-t19.*t267.*(3.9e1./2.0)-t19.*t269.*(3.9e1./2.0)+t11.*t281.*2.0-t19.*t275.*6.0+t71.*t225.*3.6e1-t71.*t227.*3.6e1+t19.*t281.*2.0+t71.*t230.*(2.7e1./2.0)-t71.*t231.*(2.7e1./2.0)-t71.*t232.*(2.7e1./2.0)-t71.*t237.*(9.0./2.0)+t71.*t238.*(9.0./2.0)+t71.*t239.*(9.0./2.0)+t71.*t240.*(9.0./2.0)+t71.*t241.*(3.0./2.0)+t11.*t331.*2.13e2-t11.*t338.*2.4e2+t19.*t331.*2.13e2-t11.*t341.*9.0e1-t11.*t345.*8.1e1-t19.*t338.*2.4e2-t19.*t341.*9.0e1+t31.*t331.*2.13e2+t11.*t352.*3.0e1-t19.*t345.*8.1e1+t11.*t356.*2.7e1+t11.*t358.*2.7e1-t31.*t338.*2.4e2+t19.*t352.*3.0e1-t31.*t341.*9.0e1+t11.*t363.*9.0+t19.*t356.*2.7e1-t31.*t345.*8.1e1+t19.*t358.*2.7e1+t19.*t363.*9.0+t31.*t352.*3.0e1-t11.*t375.*3.0+t31.*t356.*2.7e1+t31.*t358.*2.7e1-t19.*t375.*3.0+t31.*t363.*9.0+t71.*t331.*(2.13e2./2.0)-t31.*t375.*3.0-t71.*t338.*(1.59e2./2.0)-t71.*t341.*(6.3e1./2.0)+t11.*t404.*2.4e2-t71.*t345.*(8.1e1./2.0)+t11.*t407.*9.0e1-t11.*t409.*(9.0./2.0)-t11.*t411.*3.0e1+t19.*t404.*2.4e2+t19.*t407.*9.0e1+t11.*t416.*7.1e2-t19.*t409.*(9.0./2.0)-t19.*t411.*3.0e1+t19.*t416.*7.1e2+t31.*t404.*2.4e2+t31.*t407.*9.0e1-t31.*t409.*(9.0./2.0)-t31.*t411.*3.0e1-t71.*t375.*(3.0./2.0)+t31.*t416.*7.1e2-t71.*t411.*(2.1e1./2.0)-t11.*t563.*(1.0./2.0)-t19.*t563.*(1.0./2.0)-t31.*t563.*(1.0./2.0)-t71.*t563.*(1.0./2.0)-t10.*t20.*t133.*2.43e2+t10.*t16.*t140.*2.43e2-t16.*t20.*t133.*2.43e2+t10.*t16.*t144.*5.4e1-t10.*t16.*t146.*3.33e2+t10.*t16.*t148.*1.11e2-t10.*t16.*t150.*1.8e1-t10.*t16.*t153.*1.08e2+t10.*t16.*t157.*1.08e2-t10.*t16.*t160.*3.6e1-t10.*t16.*t162.*3.6e1+t10.*t16.*t194.*3.0+t10.*t16.*t223.*8.1e1+t10.*t16.*t225.*1.44e2-t10.*t16.*t227.*1.44e2-t10.*t20.*t224.*8.1e1+t10.*t20.*t225.*1.44e2+t10.*t16.*t230.*5.4e1-t10.*t16.*t231.*5.4e1-t10.*t20.*t227.*1.44e2+t10.*t20.*t230.*5.4e1-t16.*t20.*t224.*8.1e1-t10.*t20.*t231.*5.4e1+t16.*t20.*t225.*1.44e2-t10.*t20.*t232.*2.7e1-t10.*t16.*t237.*1.8e1-t16.*t20.*t227.*1.44e2+t16.*t20.*t230.*5.4e1+t10.*t16.*t241.*3.0-t10.*t20.*t237.*1.8e1-t16.*t20.*t231.*5.4e1+t10.*t20.*t238.*1.8e1-t16.*t20.*t232.*2.7e1+t10.*t20.*t239.*9.0+t10.*t20.*t240.*9.0+t10.*t20.*t241.*3.0-t10.*t16.*t247.*7.47e2-t16.*t20.*t237.*1.8e1+t16.*t20.*t238.*1.8e1+t16.*t20.*t239.*9.0+t16.*t20.*t240.*9.0+t16.*t20.*t241.*3.0+t10.*t16.*t258.*1.21e2+t10.*t51.*t225.*7.2e1-t10.*t51.*t227.*7.2e1+t10.*t51.*t230.*2.7e1-t10.*t51.*t231.*2.7e1+t16.*t51.*t225.*7.2e1-t10.*t16.*t267.*3.9e1-t10.*t51.*t232.*2.7e1-t16.*t51.*t227.*7.2e1-t10.*t16.*t269.*3.9e1+t20.*t51.*t225.*7.2e1+t16.*t51.*t230.*2.7e1-t10.*t51.*t237.*9.0-t16.*t51.*t231.*2.7e1-t20.*t51.*t227.*7.2e1+t10.*t51.*t238.*9.0-t16.*t51.*t232.*2.7e1+t10.*t51.*t239.*9.0-t10.*t16.*t275.*1.2e1+t10.*t51.*t240.*9.0+t20.*t51.*t230.*2.7e1+t10.*t51.*t241.*3.0-t20.*t51.*t231.*2.7e1-t20.*t51.*t232.*2.7e1-t16.*t51.*t237.*9.0+t16.*t51.*t238.*9.0+t16.*t51.*t239.*9.0+t10.*t16.*t281.*4.0+t16.*t51.*t240.*9.0+t16.*t51.*t241.*3.0-t20.*t51.*t237.*9.0+t20.*t51.*t238.*9.0+t20.*t51.*t239.*9.0+t20.*t51.*t240.*9.0+t20.*t51.*t241.*3.0+t10.*t16.*t331.*4.26e2+t10.*t20.*t331.*4.26e2-t10.*t16.*t338.*4.8e2-t10.*t16.*t341.*1.8e2+t16.*t20.*t331.*4.26e2-t10.*t20.*t338.*4.8e2-t10.*t16.*t345.*1.62e2-t10.*t20.*t341.*1.8e2-t16.*t20.*t338.*4.8e2-t10.*t20.*t345.*1.62e2-t16.*t20.*t341.*1.8e2+t10.*t16.*t352.*6.0e1-t16.*t20.*t345.*1.62e2+t10.*t16.*t356.*5.4e1+t10.*t20.*t352.*6.0e1+t10.*t16.*t358.*5.4e1+t10.*t20.*t356.*5.4e1+t10.*t20.*t358.*5.4e1+t16.*t20.*t352.*6.0e1+t10.*t16.*t363.*1.8e1+t10.*t51.*t331.*2.13e2+t16.*t20.*t356.*5.4e1+t10.*t20.*t363.*1.8e1+t16.*t20.*t358.*5.4e1+t16.*t51.*t331.*2.13e2-t10.*t51.*t338.*1.59e2+t16.*t20.*t363.*1.8e1-t10.*t16.*t375.*6.0-t10.*t51.*t341.*6.3e1+t20.*t51.*t331.*2.13e2-t10.*t20.*t375.*6.0-t16.*t51.*t338.*1.59e2-t10.*t51.*t345.*8.1e1-t16.*t51.*t341.*6.3e1-t20.*t51.*t338.*1.59e2-t16.*t20.*t375.*6.0-t16.*t51.*t345.*8.1e1-t20.*t51.*t341.*6.3e1-t20.*t51.*t345.*8.1e1+t10.*t16.*t404.*4.8e2+t10.*t16.*t407.*1.8e2+t10.*t20.*t404.*4.8e2-t10.*t16.*t409.*9.0-t10.*t51.*t375.*3.0-t10.*t16.*t411.*6.0e1+t10.*t20.*t407.*1.8e2-t10.*t20.*t409.*9.0+t16.*t20.*t404.*4.8e2-t10.*t20.*t411.*6.0e1+t10.*t16.*t416.*1.42e3-t16.*t51.*t375.*3.0+t16.*t20.*t407.*1.8e2-t16.*t20.*t409.*9.0+t10.*t20.*t416.*1.42e3-t20.*t51.*t375.*3.0-t16.*t20.*t411.*6.0e1+t16.*t20.*t416.*1.42e3-t10.*t51.*t411.*2.1e1-t16.*t51.*t411.*2.1e1-t20.*t51.*t411.*2.1e1-t10.*t16.*t563-t10.*t20.*t563-t16.*t20.*t563-t10.*t51.*t563-t16.*t51.*t563-t20.*t51.*t563).*-6.0;t329.*(FN.*-6.55e4+t27.*1.7878725e5+t28.*1.5671475e5-t77.*5.370975e4-t79.*1.986525e4+t83.*6.62175e3+t85.*6.62175e3-t98.*7.3575e2+t108.*6.62175e3+t109.*6.62175e3+t110.*6.62175e3+t111.*2.20725e3+t113.*4.2305625e5+t114.*1.6112925e5-t116.*5.959575e4-t118.*5.959575e4-t120.*5.2974e4-t122.*5.2974e4-t124.*1.986525e4-t126.*1.986525e4-t128.*1.986525e4+FN.*t27.*2.025e4+FN.*t28.*1.665e4-FN.*t79.*2.25e3+FN.*t111.*4.5e2+FN.*t114.*3.285e4-FN.*t124.*4.05e3-FN.*t126.*4.05e3-FN.*t128.*4.05e3+T2.*t171.*3.285e4+T2.*t173.*1.215e4+T2.*t175.*1.215e4+T2.*t177.*9.45e3+T2.*t179.*9.45e3-T2.*t196.*4.05e3-T2.*t199.*4.05e3-T2.*t202.*4.05e3-T2.*t205.*1.35e3+T2.*t214.*4.5e2-T2.*t251.*1.35e3-T2.*t261.*7.395e4+T2.*t333.*9.0e2-T3.*t333.*9.0e2-T2.*t366.*6.165e4+T3.*t366.*6.165e4+T2.*t378.*1.215e4-T3.*t378.*1.215e4+T2.*t381.*8.1e3-T3.*t381.*8.1e3+T2.*t384.*8.1e3-T3.*t384.*8.1e3-T2.*t397.*1.35e3+T3.*t397.*1.35e3+T2.*t431.*5.205e4-T3.*t431.*5.205e4-T2.*t440.*8.1e3+T3.*t440.*8.1e3-T2.*t442.*6.75e3+T3.*t442.*6.75e3-T2.*t444.*6.75e3+T3.*t444.*6.75e3+T3.*t506.*1.35e3-T4.*t506.*1.35e3-T3.*t509.*4.05e3+T4.*t509.*4.05e3+T3.*t511.*2.7e3-T4.*t511.*2.7e3+T3.*t557.*5.4e3-T4.*t557.*5.4e3-T3.*t565.*4.5e2+T4.*t565.*4.5e2-T3.*t577.*1.215e4+T4.*t577.*1.215e4+T3.*t579.*2.43e4-T4.*t579.*2.43e4-T3.*t582.*1.62e4+T4.*t582.*1.62e4+T4.*t619.*4.05e3-T4.*t621.*1.215e4-T4.*t623.*3.6e3-T4.*t631.*3.0e2-T4.*t642.*4.5e2+T4.*t643.*5.4e3+T4.*t644.*8.1e3-T4.*t645.*1.35e3+t11.*t624.*2.2575e4-t11.*t626.*1.0e2+t11.*t627.*2.025e3+t11.*t628.*2.7e3-t11.*t629.*2.7e3-t11.*t630.*2.25e2+t11.*t632.*4.5e2+t19.*t624.*2.2575e4-t19.*t626.*1.0e2+t19.*t627.*2.025e3+t19.*t628.*2.7e3+t11.*t637.*7.5e1-t19.*t629.*2.7e3+t11.*t638.*4.5e2-t19.*t630.*2.25e2+t11.*t639.*1.35e3+t11.*t640.*2.25e2+t19.*t632.*4.5e2-t11.*t641.*7.5e1+t19.*t637.*7.5e1+t11.*t646.*1.3225e4+t19.*t638.*4.5e2-t31.*t626.*1.0e2-t11.*t647.*2.025e3+t19.*t639.*1.35e3+t11.*t648.*8.1e3+t19.*t640.*2.25e2+t11.*t649.*5.4e3-t19.*t641.*7.5e1-t11.*t650.*1.35e3-t11.*t651.*1.575e3-t11.*t652.*1.575e3+t31.*t632.*4.5e2+t11.*t653.*6.75e2+t11.*t654.*2.025e3+t19.*t646.*1.3225e4+t11.*t655.*3.0e2-t19.*t647.*2.025e3+t11.*t656.*2.25e2+t19.*t648.*8.1e3-t11.*t657.*6.75e2+t19.*t649.*5.4e3+t31.*t637.*7.5e1-t11.*t658.*4.5e2-t19.*t650.*1.35e3+t31.*t638.*4.5e2+t11.*t659.*1.5e2-t19.*t651.*1.575e3+t31.*t639.*1.35e3-t19.*t652.*1.575e3+t31.*t640.*2.25e2+t19.*t653.*6.75e2-t31.*t641.*7.5e1+t19.*t654.*2.025e3+t19.*t655.*3.0e2+t19.*t656.*2.25e2-t19.*t657.*6.75e2-t19.*t658.*4.5e2+t19.*t659.*1.5e2-t31.*t647.*2.025e3+t31.*t648.*8.1e3+t31.*t649.*5.4e3+t31.*t653.*6.75e2+t31.*t654.*2.025e3+t31.*t655.*3.0e2+t31.*t656.*2.25e2-t31.*t657.*6.75e2-t31.*t658.*4.5e2-t71.*t626.*1.0e2+t71.*t637.*7.5e1+t71.*t638.*4.5e2+t71.*t639.*1.35e3+t71.*t640.*2.25e2+t71.*t653.*6.75e2+t71.*t654.*2.025e3+t71.*t655.*3.0e2+t11.*sin(t2).*7.3925e4-t11.*sin(t170).*5.475e3-t11.*sin(t172).*1.0125e4-t11.*sin(t174).*1.0125e4-t11.*sin(t176).*9.225e3-t11.*sin(t178).*9.225e3+t11.*sin(t195).*6.75e2+t11.*sin(t198).*6.75e2+t11.*sin(t201).*6.75e2+t11.*sin(t204).*1.125e3-t11.*sin(t213).*7.5e1-t11.*sin(t250).*1.125e3+t10.*t16.*t624.*4.515e4-t10.*t16.*t626.*2.0e2+t10.*t16.*t627.*4.05e3+t10.*t16.*t628.*5.4e3-t10.*t16.*t629.*5.4e3-t10.*t16.*t630.*4.5e2-t10.*t20.*t626.*2.0e2+t10.*t16.*t632.*9.0e2+t10.*t20.*t632.*9.0e2-t16.*t20.*t626.*2.0e2+t10.*t16.*t637.*1.5e2+t10.*t16.*t638.*9.0e2+t10.*t16.*t639.*2.7e3+t10.*t16.*t640.*4.5e2-t10.*t16.*t641.*1.5e2+t10.*t20.*t637.*1.5e2+t10.*t20.*t638.*9.0e2+t16.*t20.*t632.*9.0e2+t10.*t20.*t639.*2.7e3+t10.*t20.*t640.*4.5e2-t10.*t20.*t641.*1.5e2+t10.*t16.*t646.*2.645e4-t10.*t16.*t647.*4.05e3+t16.*t20.*t637.*1.5e2+t10.*t16.*t648.*1.62e4+t16.*t20.*t638.*9.0e2+t10.*t16.*t649.*1.08e4+t16.*t20.*t639.*2.7e3-t10.*t16.*t650.*2.7e3+t16.*t20.*t640.*4.5e2-t10.*t16.*t651.*3.15e3-t10.*t20.*t647.*4.05e3-t16.*t20.*t641.*1.5e2-t10.*t16.*t652.*3.15e3+t10.*t20.*t648.*1.62e4+t10.*t16.*t653.*1.35e3+t10.*t20.*t649.*1.08e4+t10.*t16.*t654.*4.05e3+t10.*t16.*t655.*6.0e2+t10.*t16.*t656.*4.5e2-t10.*t16.*t657.*1.35e3+t10.*t20.*t653.*1.35e3-t16.*t20.*t647.*4.05e3-t10.*t16.*t658.*9.0e2+t10.*t20.*t654.*4.05e3+t16.*t20.*t648.*1.62e4+t10.*t16.*t659.*3.0e2+t10.*t20.*t655.*6.0e2+t16.*t20.*t649.*1.08e4+t10.*t20.*t656.*4.5e2-t10.*t20.*t657.*1.35e3-t10.*t51.*t626.*2.0e2-t10.*t20.*t658.*9.0e2+t16.*t20.*t653.*1.35e3+t16.*t20.*t654.*4.05e3+t16.*t20.*t655.*6.0e2+t16.*t20.*t656.*4.5e2-t16.*t20.*t657.*1.35e3-t16.*t51.*t626.*2.0e2-t16.*t20.*t658.*9.0e2-t20.*t51.*t626.*2.0e2+t10.*t51.*t637.*1.5e2+t10.*t51.*t638.*9.0e2+t10.*t51.*t639.*2.7e3+t10.*t51.*t640.*4.5e2+t16.*t51.*t637.*1.5e2+t16.*t51.*t638.*9.0e2+t16.*t51.*t639.*2.7e3+t16.*t51.*t640.*4.5e2+t20.*t51.*t637.*1.5e2+t20.*t51.*t638.*9.0e2+t20.*t51.*t639.*2.7e3+t20.*t51.*t640.*4.5e2+t10.*t51.*t653.*1.35e3+t10.*t51.*t654.*4.05e3+t10.*t51.*t655.*6.0e2+t16.*t51.*t653.*1.35e3+t16.*t51.*t654.*4.05e3+t16.*t51.*t655.*6.0e2+t20.*t51.*t653.*1.35e3+t20.*t51.*t654.*4.05e3+t20.*t51.*t655.*6.0e2-6.234255e5).*(1.0./2.5e1)];
